simulink model "AxleSplitHEVv6_modif4"  (R2017a)
settings: Solver=ode5  StartTime=0.0  StopTime=400  FixedStep=hev_dt  MaxStep=0.01  RelTol=1e-3  AbsTol=1e-3  EnableMultiTasking=on
PostLoadFcn:
  | load('AxelSplitHEVv4_NEDC_18_06_15.mat')
values from neighbouring files (symbols this model uses):
  cmd_equivalent_conso_coef = 0.11126984    [AxelSplitHEVv4_NEDC_18_06_15.mat]
  cmd_qmax = 42    [AxelSplitHEVv4_NEDC_18_06_15.mat]
  cmd_specific_volume_l_per_g = 0.00133333333333    [AxelSplitHEVv4_NEDC_18_06_15.mat]
  dri_cycle_speed_sp = [0 0 0 4.16666667 4.16666667 2.777777778 0 0 0 4.166666667 4.166666667 8.88888889 ... (135 elements, 135x1)]    [AxelSplitHEVv4_NEDC_18_06_15.mat]
  dri_cycle_speed_time = [0 6 11 15 23 25 28 44 49 54 56 61 ... (135 elements, 135x1)]    [AxelSplitHEVv4_NEDC_18_06_15.mat]
  dri_gbx_sp = [0 1 0 1 2 0 1 2 3 2 0 1 ... (52 elements, 52x1)]    [AxelSplitHEVv4_NEDC_18_06_15.mat]
  dri_gbx_time = [0 11 25 49 55 93 117 123 134 177 185 206 ... (52 elements, 52x1)]    [AxelSplitHEVv4_NEDC_18_06_15.mat]
  dri_ki = 24.5    [AxelSplitHEVv4_NEDC_18_06_15.mat]
  dri_kp = 609    [AxelSplitHEVv4_NEDC_18_06_15.mat]
  fa_clu_pos = [1 1 0.7 0.5 0.3 0 0]    [AxelSplitHEVv4_NEDC_18_06_15.mat]
  fa_clu_pv = [0 0.1 0.3 0.5 0.7 0.9 1]    [AxelSplitHEVv4_NEDC_18_06_15.mat]
  fa_conso_idle = 0.153611111111    [AxelSplitHEVv4_NEDC_18_06_15.mat]
  fa_conso_speed = [200 300 400 500 600 700 800 900 1000 1100 1200 1300 ... (56 elements, 1x56)]    [AxelSplitHEVv4_NEDC_18_06_15.mat]
  fa_conso_torque = [0 6.66666666667 13.3333333333 20 26.6666666667 33.3333333333 40 46.6666666667 53.3333333333 60 66.6666666667 73.3333333333 ... (43 elements, 1x43)]    [AxelSplitHEVv4_NEDC_18_06_15.mat]
  fa_delta_derating = 500    [AxelSplitHEVv4_NEDC_18_06_15.mat]
  fa_differential_ratio = FDR.fa_differential_ratio    [Algorithme_eff.m]    (also in AxelSplitHEVv4_NEDC_18_06_15.mat = 3.72; fa_differential_ratio.mat = 3.72)
  fa_fuel_consumption = [nan nan nan nan nan nan nan nan nan nan nan nan ... (2408 elements, 43x56)]    [AxelSplitHEVv4_NEDC_18_06_15.mat]    (also in Curve_fitting_conso.m = fa_fuel_consumption/max(max(fa_fuel_consumption)))
  fa_gearbox_efficiency = 0.92    [AxelSplitHEVv4_NEDC_18_06_15.mat]
  fa_gearbox_ratio = FGR.fa_gearbox_ratio    [Algorithme_eff.m]    (also in AxelSplitHEVv4_NEDC_18_06_15.mat = [0 3.98 2.21 1.47 1.1 0.89 0.75]; fa_gearbox_ratio.mat = [0 3.98 2.21 1.47 1.1 0.89 0.75])
  fa_high_derating_point = 5700    [AxelSplitHEVv4_NEDC_18_06_15.mat]
  fa_ice_inertia = 0.058    [AxelSplitHEVv4_NEDC_18_06_15.mat]
  fa_kp_idle_tr_off = 0.116198282851    [AxelSplitHEVv4_NEDC_18_06_15.mat]
  fa_kp_idle_tr_on = [1 0.8653 2.8063 6.3428 11.3274 17.3036 24.3665]    [AxelSplitHEVv4_NEDC_18_06_15.mat]
  fa_low_derating_point = 4000    [AxelSplitHEVv4_NEDC_18_06_15.mat]
  fa_max_tq_clu = 206    [AxelSplitHEVv4_NEDC_18_06_15.mat]
  fa_max_tq_ice = [0 220 233.333333333 240 246.666666667 253.333333333 253.333333333 253.333333333 260 260 266.666666667 266.666666667 ... (52 elements, 1x52)]    [AxelSplitHEVv4_NEDC_18_06_15.mat]
  fa_n_ice = [0 20 250 850 1000 1250 1500 1750 2000 2250 2500 3000 ... (18 elements, 1x18)]    [AxelSplitHEVv4_NEDC_18_06_15.mat]
  fa_starter_rpm = [0 10 20 30 40 50 60 70 80 90 100 110 ... (101 elements, 1x101)]    [AxelSplitHEVv4_NEDC_18_06_15.mat]
  fa_starter_tq = [24 24 24 24 23.3333333333 23.3333333333 23.3333333333 22.6666666667 22.6666666667 22 21.3333333333 20.6666666667 ... (101 elements, 1x101)]    [AxelSplitHEVv4_NEDC_18_06_15.mat]
  fa_tau_ice = 0.0333    [AxelSplitHEVv4_NEDC_18_06_15.mat]
  fa_taui_idle_tr_off = 0.0820482966067    [AxelSplitHEVv4_NEDC_18_06_15.mat]
  fa_taui_idle_tr_on = 0.194086623254    [AxelSplitHEVv4_NEDC_18_06_15.mat]
  fa_tq_loss = [0 -11 -10 -9 -9 -10 -11 -11 -12 -13 -14 -15 ... (18 elements, 1x18)]    [AxelSplitHEVv4_NEDC_18_06_15.mat]
  fa_tq_max_speed = [200 700 800 900 1000 1100 1200 1300 1400 1500 1600 1700 ... (52 elements, 1x52)]    [AxelSplitHEVv4_NEDC_18_06_15.mat]
  hev_dt = 0.01    [AxelSplitHEVv4_NEDC_18_06_15.mat]
  pla_csat = 1.2    [AxelSplitHEVv4_NEDC_18_06_15.mat]
  pla_equivalent_weight = 1250    [AxelSplitHEVv4_NEDC_18_06_15.mat]
  pla_f = 0.0035272    [AxelSplitHEVv4_NEDC_18_06_15.mat]
  pla_k = 0.0002318    [AxelSplitHEVv4_NEDC_18_06_15.mat]
  pla_kaero = 0.52992    [AxelSplitHEVv4_NEDC_18_06_15.mat]
  pla_max_f_brakes = 1000    [AxelSplitHEVv4_NEDC_18_06_15.mat]
  pla_wheel_radius = 0.314    [AxelSplitHEVv4_NEDC_18_06_15.mat]
  ra_electrical_machine_efficiency = [nan nan nan nan nan nan nan 91.3 91.3 91.3 91.5 91.3 ... (777 elements, 37x21)]    [AxelSplitHEVv4_NEDC_18_06_15.mat]
  ra_electrical_machine_speed = [-12000 -10800 -9600 -8400 -7200 -6000 -4800 -3600 -2400 -1200 0 1200 ... (21 elements, 1x21)]    [AxelSplitHEVv4_NEDC_18_06_15.mat]
  ra_electrical_machine_tau = 0.1    [AxelSplitHEVv4_NEDC_18_06_15.mat]
  ra_electrical_machine_torque = [-79.6460176991 -75.2212389381 -70.796460177 -66.3716814159 -61.9469026549 -57.5221238938 -53.0973451327 -48.6725663717 -44.2477876106 -39.8230088496 -35.3982300885 -30.9734513274 ... (37 elements, 1x37)]    [AxelSplitHEVv4_NEDC_18_06_15.mat]
  ra_em_max_tq = [39.8230088496 44.2477876106 53.0973451327 57.5221238938 70.796460177 79.6460176991 79.6460176991 79.6460176991 79.6460176991 79.6460176991 79.6460176991 79.6460176991 ... (21 elements, 1x21)]    [AxelSplitHEVv4_NEDC_18_06_15.mat]
  ra_em_min_tq = [-39.8230088496 -44.2477876106 -53.0973451327 -57.5221238938 -70.796460177 -79.6460176991 -79.6460176991 -79.6460176991 -79.6460176991 -79.6460176991 -79.6460176991 -79.6460176991 ... (21 elements, 1x21)]    [AxelSplitHEVv4_NEDC_18_06_15.mat]
  ra_transmission_efficiency = 0.92    [AxelSplitHEVv4_NEDC_18_06_15.mat]
  reducteur = 2    [Main_modif.m]
  syse_aux_current = 33.3    [AxelSplitHEVv4_NEDC_18_06_15.mat]
  syse_aux_voltage = 12    [AxelSplitHEVv4_NEDC_18_06_15.mat]
  syse_bat_nominal_capacity_as = 151200    [AxelSplitHEVv4_NEDC_18_06_15.mat]
  syse_cdl = 5000    [AxelSplitHEVv4_NEDC_18_06_15.mat]
  syse_dcdc_efficency = [78 89.6 92.5 95.2 95 94.6]    [AxelSplitHEVv4_NEDC_18_06_15.mat]
  syse_dcdc_in_power = [54 135 202 405 1485 2000]    [AxelSplitHEVv4_NEDC_18_06_15.mat]
  syse_electrical_machine_torque_vs_power_speed_nneg = [38.4209635438 42.3166718474 53.0973451327 53.8788373627 63.500986907 77.9700595469 78.3175021924 76.9635177026 72.2987813984 47.9837613501 38.4209635438 42.3166718474 ... (220 elements, 10x22)]    [AxelSplitHEVv4_NEDC_18_06_15.mat]
  syse_electrical_machine_torque_vs_power_speed_npos = [-72.2987813984 -76.9635177026 -78.3175021924 -77.9700595469 -63.500986907 -53.8788373627 -53.0973451327 -42.3166718474 -38.4209635438 -72.2987813984 -76.9635177026 -78.3175021924 ... (198 elements, 9x22)]    [AxelSplitHEVv4_NEDC_18_06_15.mat]
  syse_em_in_power = [-49.1089315336 -44.1089315336 -39.1089315336 -34.1089315336 -29.1089315336 -24.1089315336 -19.1089315336 -14.1089315336 -9.10893153364 -4.10893153364 0.891068466363 5.89106846636 ... (22 elements, 1x22)]    [AxelSplitHEVv4_NEDC_18_06_15.mat]
  syse_max_charge_current = [8.4 8.4 42 92.4 92.4 92.4 92.4 92.4 79.8 42 21 4.2]    [AxelSplitHEVv4_NEDC_18_06_15.mat]
  syse_max_discharge_current = [42 42 79.8 159.6 180.6 180.6 180.6 180.6 180.6 180.6 180.6 180.6]    [AxelSplitHEVv4_NEDC_18_06_15.mat]
  syse_nb_cell = 52    [AxelSplitHEVv4_NEDC_18_06_15.mat]
  syse_rdl = 0.004    [AxelSplitHEVv4_NEDC_18_06_15.mat]
  syse_rser = 0.002    [AxelSplitHEVv4_NEDC_18_06_15.mat]
  syse_soc_current_limits = [0 10 20 20.1 30 40 50 60 70 80 90 100]    [AxelSplitHEVv4_NEDC_18_06_15.mat]
  syse_soc_initial = 0.8    [AxelSplitHEVv4_NEDC_18_06_15.mat]
  syse_soc_ocv = [0 5 10 20 40 50 60 70 80 90 100]    [AxelSplitHEVv4_NEDC_18_06_15.mat]
  syse_vocv = [2.5 3.2135 3.5127 3.66 3.7771 3.8181 3.8686 3.8978 3.9429 4.0006 4.198]    [AxelSplitHEVv4_NEDC_18_06_15.mat]
undefined symbols (not defined in the file or in its folder): DiscIntNeverNeededParam
libraries: simulink x23, simulink_extras x1
(part 3 of 3)

== system AxleSplitHEVv6_modif4/HEV model/Command/Torque repartition/Optimization Algorithm /Sfunction: Optimization Algorithm 32bits ==
  T : Inport
  V : Inport  Port=2
  Tmax_elec : Inport  Port=3
  Tmin_elec : Inport  Port=4
  Tmax_therm : Inport  Port=5
  Tmin_therm : Inport  Port=6
  GBX : Inport  Port=7
  SOC : Inport  Port=8
  MATLAB Function: Optimization Algorithm_sfcn : S-Function  FunctionName=MATLAB_sf  SFunctionModules=""  SFunctionDeploymentMode=off  EnableBusSupport=off  mask{rtw_sf_name=MATLAB_sf, showVar=off}
      mask prompts: rtw_sf_name "Simulink:masks:GenSFuncName_MP"; showVar "Simulink:masks:GenSFuncShowModuleList_MP"
      mask help: Simulink:masks:GenSFuncDesc_MD
      mask init:
      | displist = '';
      | if ~strcmp(get_param(gcb, 'FunctionName'), rtw_sf_name);
      |   set_param(gcb, 'FunctionName', rtw_sf_name);
      | end
      | % Check if we are generating code
      | rtw_mode = false;
      | if strcmpi(get_param(bdroot(gcb),'SimulationStatus'),'Initializing')
      | 	rtw_mode = strcmpi(get_param(bdroot(gcb),'BuildingRTWCode'),'on') && ...
      | 		~strcmpi(get_param(bdroot(gcb),'TargetStyle'),'SimulationTarget');
      | end
      | if showVar || rtw_mode
      | 	if exist('rtwsfunc') == 2 | exist('rtwsfunc') == 6
      | 		tmplist = rtwsfunc(rtw_sf_name,gcb);
      | 		tmplist = DAStudio.message('Simulink:masks:GenSFuncListOfModules_IC', tmplist);
      | 	elseif showVar
      | 		tmplist1 = DAStudio.message('Simulink:masks:GenSFuncListOfModules_IC', '');
      |         tmplist2 = DAStudio.message('Simulink:masks:GenSFuncNotLicensed_IC');
      |         tmplist = [tmplist1 tmplist2];
      |  	end
      | end
      | if showVar
      |   displist = tmplist;
      | end
      settings: CopyFcn=|
      | if ~strcmp(get_param(gcb,'Linkstatus'),'none') && ...
      | ~strcmp(get_param(gcb,'Linkstatus'),'implicit')
      |   set_param(gcb,'LinkStatus','none');
      | end
      mask Help: eval('feval(''rtwprivate'',''rtwhelpview'',''rtw_sfcn_block'')');
      mask Display:
      | port_label('input',1,'T');
      | port_label('input',2,'V');
      | port_label('input',3,'Tmax_elec');
      | port_label('input',4,'Tmin_elec');
      | port_label('input',5,'Tmax_therm');
      | port_label('input',6,'Tmin_therm');
      | port_label('input',7,'GBX');
      | port_label('input',8,'SOC');
      | port_label('output',1,'alpha_opt');
  __InputSSForSFun__ : Subsystem
  __OutputSSForSFun__ : Subsystem
  alpha_opt : Outport
  wires:
  T/1 -> __InputSSForSFun__/1(T)
  V/1 -> __InputSSForSFun__/2(V)
  Tmax_elec/1 -> __InputSSForSFun__/3(Tmax_elec)
  Tmin_elec/1 -> __InputSSForSFun__/4(Tmin_elec)
  Tmax_therm/1 -> __InputSSForSFun__/5(Tmax_therm)
  Tmin_therm/1 -> __InputSSForSFun__/6(Tmin_therm)
  GBX/1 -> __InputSSForSFun__/7(GBX)
  SOC/1 -> __InputSSForSFun__/8(SOC)
  __InputSSForSFun__/1(__UniqueOutportName__1__) -> MATLAB Function: Optimization Algorithm_sfcn/1
  __InputSSForSFun__/2(__UniqueOutportName__2__) -> MATLAB Function: Optimization Algorithm_sfcn/2
  __InputSSForSFun__/3(__UniqueOutportName__3__) -> MATLAB Function: Optimization Algorithm_sfcn/3
  __InputSSForSFun__/4(__UniqueOutportName__4__) -> MATLAB Function: Optimization Algorithm_sfcn/4
  __InputSSForSFun__/5(__UniqueOutportName__5__) -> MATLAB Function: Optimization Algorithm_sfcn/5
  __InputSSForSFun__/6(__UniqueOutportName__6__) -> MATLAB Function: Optimization Algorithm_sfcn/6
  __InputSSForSFun__/7(__UniqueOutportName__7__) -> MATLAB Function: Optimization Algorithm_sfcn/7
  __InputSSForSFun__/8(__UniqueOutportName__8__) -> MATLAB Function: Optimization Algorithm_sfcn/8
  MATLAB Function: Optimization Algorithm_sfcn/1 -> __OutputSSForSFun__/1(__UniqueInportName__1__)
  __OutputSSForSFun__/1(alpha_opt) -> alpha_opt/1

== system AxleSplitHEVv6_modif4/HEV model/Electrical system/Lithium-Ion Battery Management System/Battery model/li-ion Battery SOC ==
  SYSE_LIION_CURRENT : Inport
  Discrete-Time Integrator : DiscreteIntegrator  IntegratorMethod=Integration: Trapezoidal  InitialConditionSource=external  SampleTime=hev_dt  LimitOutput=on  UpperSaturationLimit=1  LowerSaturationLimit=0  ICPrevOutput=DiscIntNeverNeededParam  ICPrevScaledInput=DiscIntNeverNeededParam
  Divide1 : Product  Inputs=/*  SampleTime=hev_dt
  Gain : Gain  Gain=-1  SampleTime=hev_dt
  Nominal capacity : Constant  Value=syse_bat_nominal_capacity_as
  syse_soc_initial : Constant  Value=syse_soc_initial
  SYSE_SOC : Outport
  wires:
  Nominal capacity/1 -> Divide1/1  "A.s"
  Discrete-Time Integrator/1 -> SYSE_SOC/1
  syse_soc_initial/1 -> Discrete-Time Integrator/2
  Divide1/1 -> Discrete-Time Integrator/1  "s"
  SYSE_LIION_CURRENT/1 -> Gain/1  "A"
  Gain/1 -> Divide1/2

== system AxleSplitHEVv6_modif4/HEV model/Electrical system/Lithium-Ion Battery Management System/Battery model/li-ion battery voltage ==
  SYSE_SOC : Inport
  SYSE_LIION_CURRENT : Inport  Port=2
  Add2 : Sum  Inputs=+--  SampleTime=hev_dt
  Discrete Transfer Fcn1 : DiscreteTransferFcn  Numerator=[(hev_dt/(2*(syse_rdl*syse_cdl)+hev_dt)) (hev_dt/(2* (syse_rdl*syse_cdl)+hev_dt))]  Denominator=[1 ((hev_dt-2*(syse_rdl*syse_cdl)))/(2*(syse_rdl*syse_cdl)+hev_dt)]  SampleTime=hev_dt
  Gain : Gain  Gain=syse_rdl  SampleTime=hev_dt
  Lookup table Vocv : Lookup_n-D  NumberOfTableDimensions=1  BreakpointsForDimension1=syse_soc_ocv/100  Table=syse_vocv  SampleTime=hev_dt  RndMeth=Simplest  InputSameDT=on
  Rser : Gain  Gain=syse_rser  SampleTime=hev_dt
  nb of cell : Gain  Gain=syse_nb_cell  SampleTime=hev_dt
  SYSE_VOLTAGE_HV : Outport
  wires:
  SYSE_LIION_CURRENT/1 -> Gain/1, Rser/1
  SYSE_SOC/1 -> Lookup table Vocv/1
  Lookup table Vocv/1 -> Add2/1
  Add2/1 -> nb of cell/1
  nb of cell/1 -> SYSE_VOLTAGE_HV/1
  Rser/1 -> Add2/2
  Discrete Transfer Fcn1/1 -> Add2/3
  Gain/1 -> Discrete Transfer Fcn1/1

== system AxleSplitHEVv6_modif4/HEV model/Front Axle/CLUTCH/Clutch0/Stuck logic ==
  FA_W_CAR_INTEGRATOR_STATE : Inport
  FA_W_CAR : Inport  Port=2
  FA_TQ_ICE : Inport  Port=3
  FA_CLU_MAX_STATIC_TORQUE : Inport  Port=4
  Abs : Abs  SampleTime=hev_dt  SaturateOnIntegerOverflow=on
  Abs1 : Abs  SampleTime=hev_dt  SaturateOnIntegerOverflow=on
  Abs2 : Abs  SampleTime=hev_dt  SaturateOnIntegerOverflow=on
  Combinatorial Logic3 : CombinatorialLogic  Description=TRUTH_TABLE_FROM_FABIEN  TruthTable=[0;1;0;0;1;1;0;1]  SampleTime=hev_dt
  Compare To Constant : simulink/Logic and Bit Operations/Compare To Constant  relop=<=  const=40  OutDataTypeStr=boolean
  Delay : Delay  DelayLength=1  SampleTime=hev_dt
  Logic : Logic  IconShape=distinctive  SampleTime=hev_dt
  Mux : Mux  Inputs=3
  Relational Operator : RelationalOperator  Operator=<=  SampleTime=hev_dt  RndMeth=Nearest  InputSameDT=on
  Relational Operator1 : RelationalOperator  Operator=<=  SampleTime=hev_dt  RndMeth=Nearest  InputSameDT=on
  Scope2 : Scope
  Sum1 : Sum  Inputs=+-  SampleTime=hev_dt  SaturateOnIntegerOverflow=on  InputSameDT=on  OutDataTypeStr=Inherit: Same as first input
  FA_CLU_STUCK : Outport
  wires:
  FA_CLU_MAX_STATIC_TORQUE/1 -> Relational Operator1/2, Relational Operator/1
  Sum1/1 -> Abs2/1
  Abs1/1 -> Relational Operator1/1
  Delay/1 -> Mux/3
  Combinatorial Logic3/1 -> Delay/1, FA_CLU_STUCK/1
  Mux/1 -> Combinatorial Logic3/1
  Abs/1 -> Relational Operator/2
  Relational Operator/1 -> Mux/2
  Logic/1 -> Mux/1
  Abs2/1 -> Compare To Constant/1
  Compare To Constant/1 -> Logic/1
  Relational Operator1/1 -> Scope2/1, Logic/2
  FA_TQ_ICE/1 -> Abs1/1, Abs/1
  FA_W_CAR_INTEGRATOR_STATE/1 -> Sum1/1
  FA_W_CAR/1 -> Sum1/2

== system AxleSplitHEVv6_modif4/HEV model/Front Axle/CLUTCH/Clutch1/Stuck logic ==
  FA_W_CAR_INTEGRATOR_STATE : Inport
  FA_W_CAR : Inport  Port=2
  FA_TQ_ICE : Inport  Port=3
  FA_CLU_MAX_STATIC_TORQUE : Inport  Port=4
  Abs : Abs  SampleTime=hev_dt  SaturateOnIntegerOverflow=on
  Abs1 : Abs  SampleTime=hev_dt  SaturateOnIntegerOverflow=on
  Abs2 : Abs  SampleTime=hev_dt  SaturateOnIntegerOverflow=on
  Combinatorial Logic3 : CombinatorialLogic  Description=TRUTH_TABLE_FROM_FABIEN  TruthTable=[0;1;0;0;1;1;0;1]  SampleTime=hev_dt
  Compare To Constant : simulink/Logic and Bit Operations/Compare To Constant  relop=<=  const=40  OutDataTypeStr=boolean
  Delay : Delay  DelayLength=1  SampleTime=hev_dt
  Logic : Logic  IconShape=distinctive  SampleTime=hev_dt
  Mux : Mux  Inputs=3
  Relational Operator : RelationalOperator  Operator=<=  SampleTime=hev_dt  RndMeth=Nearest  InputSameDT=on
  Relational Operator1 : RelationalOperator  Operator=<=  SampleTime=hev_dt  RndMeth=Nearest  InputSameDT=on
  Scope2 : Scope
  Sum1 : Sum  Inputs=+-  SampleTime=hev_dt  SaturateOnIntegerOverflow=on  InputSameDT=on  OutDataTypeStr=Inherit: Same as first input
  FA_CLU_STUCK : Outport
  wires:
  FA_CLU_MAX_STATIC_TORQUE/1 -> Relational Operator1/2, Relational Operator/1
  Sum1/1 -> Abs2/1
  Abs1/1 -> Relational Operator1/1
  Delay/1 -> Mux/3
  Combinatorial Logic3/1 -> Delay/1, FA_CLU_STUCK/1
  Mux/1 -> Combinatorial Logic3/1
  Abs/1 -> Relational Operator/2
  Relational Operator/1 -> Mux/2
  Logic/1 -> Mux/1
  Abs2/1 -> Compare To Constant/1
  Compare To Constant/1 -> Logic/1
  Relational Operator1/1 -> Scope2/1, Logic/2
  FA_TQ_ICE/1 -> Abs1/1, Abs/1
  FA_W_CAR_INTEGRATOR_STATE/1 -> Sum1/1
  FA_W_CAR/1 -> Sum1/2

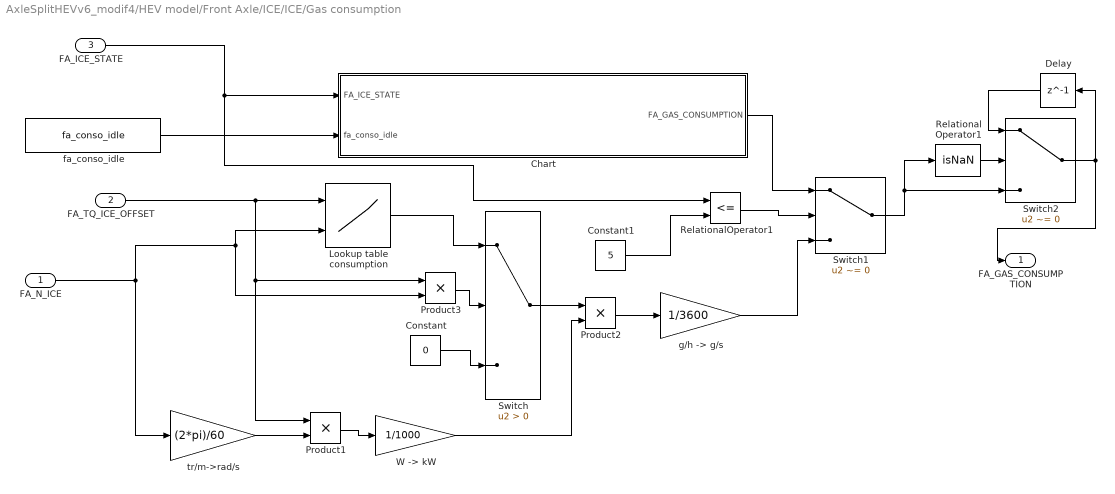
== system AxleSplitHEVv6_modif4/HEV model/Front Axle/ICE/ICE/Gas consumption ==
  FA_N_ICE : Inport
  FA_TQ_ICE_OFFSET : Inport  Port=2
  FA_ICE_STATE : Inport  Port=3
  Chart : Stateflow chart  TreatAsAtomicUnit=on
  Constant : Constant  Value=0
  Constant1 : Constant  Value=5
  Delay : Delay  DelayLength=1  SampleTime=hev_dt
  Lookup table consumption : Lookup_n-D  BreakpointsForDimension1=fa_conso_torque  BreakpointsForDimension2=fa_conso_speed  Table=fa_fuel_consumption  ExtrapMethod=Clip  UseLastTableValue=on  SampleTime=hev_dt  RndMeth=Simplest  InputSameDT=on
  Product1 : Product  SampleTime=hev_dt  RndMeth=Zero
  Product2 : Product  SampleTime=hev_dt  RndMeth=Zero
  Product3 : Product  SampleTime=hev_dt  RndMeth=Zero
  Relational Operator1 : RelationalOperator  Operator=isNaN  OutDataTypeStr=boolean  SampleTime=hev_dt  RndMeth=Nearest
  RelationalOperator1 : RelationalOperator  Operator=<=  OutDataTypeStr=boolean  SampleTime=hev_dt  RndMeth=Nearest
  Switch : Switch  Criteria=u2 > Threshold  SampleTime=hev_dt
  Switch1 : Switch  Criteria=u2 ~= 0  SampleTime=hev_dt
  Switch2 : Switch  Criteria=u2 ~= 0  SampleTime=hev_dt
  "W -> kW" : Gain  Gain=1/1000  SampleTime=hev_dt
  fa_conso_idle : Constant  Value=fa_conso_idle
  "g/h -> g/s" : Gain  Gain=1/3600  SampleTime=hev_dt
  tr/m->rad/s : Gain  Gain=(2*pi)/60  SampleTime=hev_dt
  FA_GAS_CONSUMPTION : Outport
  wires:
  Lookup table consumption/1 -> Switch/1
  Switch/1 -> Product2/1
  Constant/1 -> Switch/3
  "W -> kW"/1 -> Product2/2
  Product1/1 -> "W -> kW"/1
  tr/m->rad/s/1 -> Product1/2
  Product2/1 -> "g/h -> g/s"/1
  FA_N_ICE/1 -> Lookup table consumption/2, Product3/2, tr/m->rad/s/1
  FA_TQ_ICE_OFFSET/1 -> Product3/1, Product1/1, Lookup table consumption/1
  Product3/1 -> Switch/2
  Switch1/1 -> Switch2/3, Relational Operator1/1
  Switch2/1 -> FA_GAS_CONSUMPTION/1, Delay/1
  Relational Operator1/1 -> Switch2/2
  Delay/1 -> Switch2/1
  FA_ICE_STATE/1 -> RelationalOperator1/1, Chart/1(FA_ICE_STATE)
  "g/h -> g/s"/1 -> Switch1/3
  Chart/1(FA_GAS_CONSUMPTION) -> Switch1/1
  Constant1/1 -> RelationalOperator1/2
  RelationalOperator1/1 -> Switch1/2
  fa_conso_idle/1 -> Chart/2(fa_conso_idle)

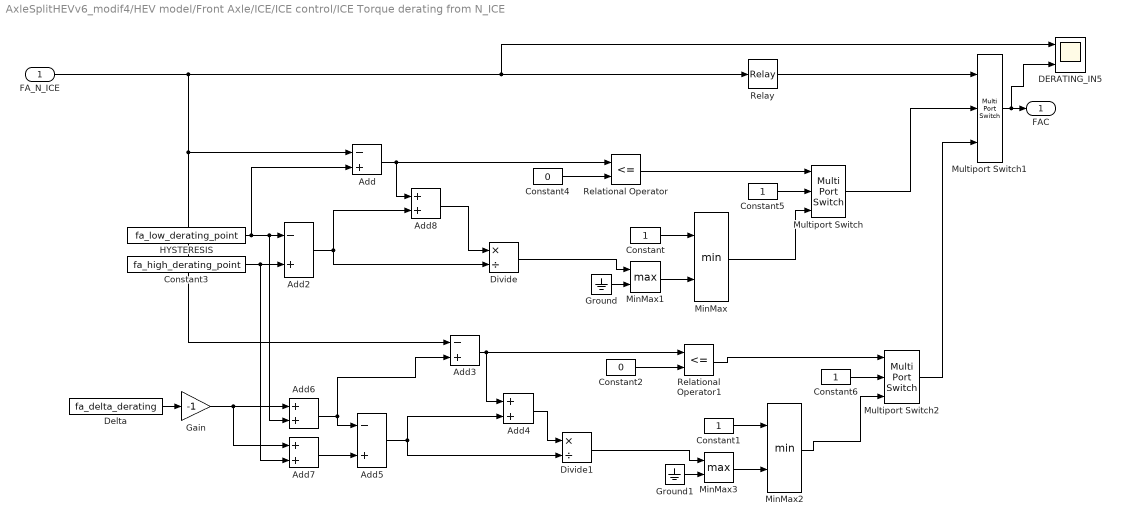
== system AxleSplitHEVv6_modif4/HEV model/Front Axle/ICE/ICE control/ICE Torque derating from N_ICE ==
  FA_N_ICE : Inport
  Add{,2..3,5} (4 alike) : Sum  Inputs=-+
  Add{4,6..8} (4 alike) : Sum
  Constant{,1,5..6} (4 alike) : Constant
  Constant2 : Constant  Value=0
  Constant3 : Constant  Value=fa_high_derating_point
  Constant4 : Constant  Value=0
  DERATING_IN5 : Scope  NumInputPorts=2
  Delta : Constant  Value=fa_delta_derating
  Divide : Product  Inputs=*/
  Divide1 : Product  Inputs=*/
  Gain : Gain  Gain=-1
  Ground : Ground
  Ground1 : Ground
  HYSTERESIS : Constant  Value=fa_low_derating_point
  MinMax : MinMax  Inputs=2
  MinMax1 : MinMax  Function=max  Inputs=2
  MinMax2 : MinMax  Inputs=2
  MinMax3 : MinMax  Function=max  Inputs=2
  Multiport Switch : MultiPortSwitch  DataPortOrder=Zero-based contiguous  Inputs=2
  Multiport Switch1 : MultiPortSwitch  DataPortOrder=Zero-based contiguous  Inputs=2
  Multiport Switch2 : MultiPortSwitch  DataPortOrder=Zero-based contiguous  Inputs=2
  Relational Operator : RelationalOperator  Operator=<=  OutDataTypeStr=boolean  RndMeth=Nearest
  Relational Operator1 : RelationalOperator  Operator=<=  OutDataTypeStr=boolean  RndMeth=Nearest
  Relay : Relay  OnSwitchValue=5750  OffSwitchValue=4900-500
  FAC : Outport
  wires:
  Gain/1 -> Add6/1, Add7/1
  Add4/1 -> Divide1/1
  Add8/1 -> Divide/1
  Add7/1 -> Add5/2
  Add6/1 -> Add3/2, Add5/1
  Constant6/1 -> Multiport Switch2/2
  MinMax2/1 -> Multiport Switch2/3
  Relational Operator1/1 -> Multiport Switch2/1
  Constant2/1 -> Relational Operator1/2
  Add3/1 -> Relational Operator1/1, Add4/1
  Divide1/1 -> MinMax3/1
  MinMax3/1 -> MinMax2/2
  Ground1/1 -> MinMax3/2
  Constant1/1 -> MinMax2/1
  FA_N_ICE/1 -> Add3/1, Add/1, Relay/1, DERATING_IN5/1
  Delta/1 -> Gain/1
  Constant3/1 -> Add2/2, Add7/2
  Multiport Switch2/1 -> Multiport Switch1/3
  HYSTERESIS/1 -> Add6/2, Add2/1, Add/2
  Multiport Switch/1 -> Multiport Switch1/2
  Constant5/1 -> Multiport Switch/2
  MinMax/1 -> Multiport Switch/3
  Relational Operator/1 -> Multiport Switch/1
  Constant4/1 -> Relational Operator/2
  Add/1 -> Add8/1, Relational Operator/1
  Relay/1 -> Multiport Switch1/1
  Divide/1 -> MinMax1/1
  MinMax1/1 -> MinMax/2
  Ground/1 -> MinMax1/2
  Constant/1 -> MinMax/1
  Multiport Switch1/1 -> FAC/1, DERATING_IN5/2
  Add2/1 -> Divide/2, Add8/2
  Add5/1 -> Divide1/2, Add4/2

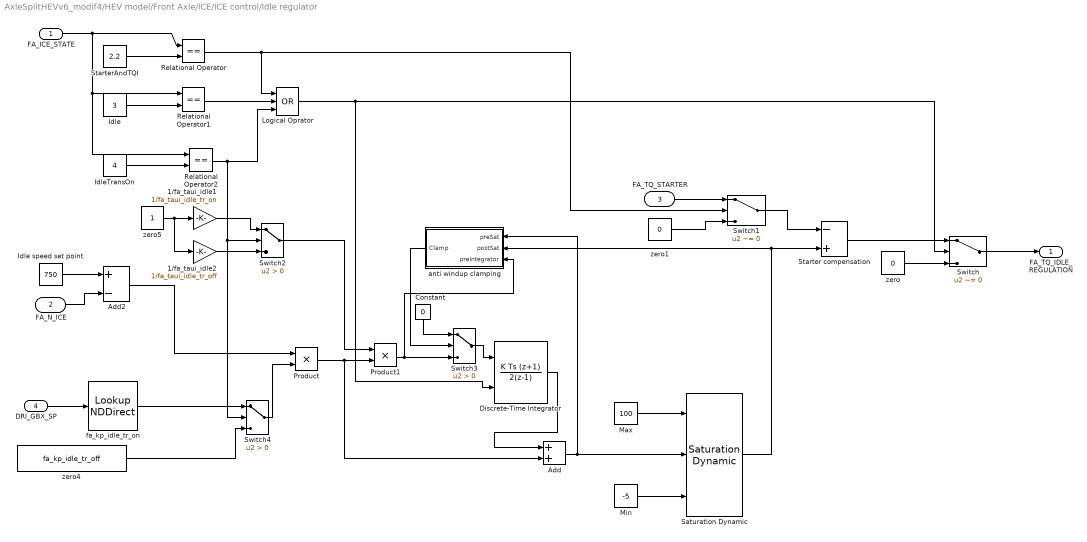
== system AxleSplitHEVv6_modif4/HEV model/Front Axle/ICE/ICE control/Idle regulator ==
  FA_ICE_STATE : Inport
  FA_N_ICE : Inport  Port=2
  FA_TQ_STARTER : Inport  Port=3
  DRI_GBX_SP : Inport  Port=4
  1/fa_taui_idle1 : Gain  Gain=1/fa_taui_idle_tr_on  SampleTime=hev_dt
  1/fa_taui_idle2 : Gain  Gain=1/fa_taui_idle_tr_off  SampleTime=hev_dt
  Add : Sum  SampleTime=hev_dt
  Add2 : Sum  Inputs=+-  SampleTime=hev_dt
  Constant : Constant  DisableCoverage=on  Value=0  OutDataTypeStr=Inherit: Inherit via back propagation  PreserveConstantTs=on
  Discrete-Time Integrator : DiscreteIntegrator  IntegratorMethod=Integration: Trapezoidal  ExternalReset=rising  SampleTime=hev_dt  ICPrevOutput=DiscIntNeverNeededParam  ICPrevScaledInput=DiscIntNeverNeededParam
  Idle : Constant  Value=3
  Idle speed set point : Constant  Value=750
  IdleTransOn : Constant  Value=4
  Logical Oprator : Logic  Operator=OR  Inputs=3  AllPortsSameDT=off  OutDataTypeStr=boolean  SampleTime=hev_dt
  Max : Constant  Value=100
  Min : Constant  Value=-5
  Product : Product  SampleTime=hev_dt  RndMeth=Zero
  Product1 : Product  SampleTime=hev_dt  RndMeth=Zero
  Relational Operator : RelationalOperator  Operator===  OutDataTypeStr=boolean  SampleTime=hev_dt  RndMeth=Nearest
  Relational Operator1 : RelationalOperator  Operator===  OutDataTypeStr=boolean  SampleTime=hev_dt  RndMeth=Nearest
  Relational Operator2 : RelationalOperator  Operator===  OutDataTypeStr=boolean  SampleTime=hev_dt  RndMeth=Nearest
  Saturation Dynamic : simulink/Discontinuities/Saturation Dynamic  OutMin=[]  OutMax=[]  OutDataTypeStr=Inherit: Same as second input  OutDataType=fixdt(1, 16)  OutScaling=2^-10  DoSatur=off
  Starter compensation : Sum  Inputs=-+  SampleTime=hev_dt
  StarterAndTQI : Constant  Value=2.2
  Switch : Switch  Criteria=u2 ~= 0  SampleTime=hev_dt
  Switch1 : Switch  Criteria=u2 ~= 0  SampleTime=hev_dt
  Switch2 : Switch  DisableCoverage=on  Criteria=u2 > Threshold  SampleTime=hev_dt  InputSameDT=on
  Switch3 : Switch  DisableCoverage=on  Criteria=u2 > Threshold  SampleTime=hev_dt  InputSameDT=on
  Switch4 : Switch  DisableCoverage=on  Criteria=u2 > Threshold  SampleTime=hev_dt  InputSameDT=on
  anti windup clamping : Subsystem
  fa_kp_idle_tr_on : LookupNDDirect  NumberOfTableDimensions=1  Table=fa_kp_idle_tr_on  SampleTime=hev_dt
  zero : Constant  Value=0
  zero1 : Constant  Value=0
  zero4 : Constant  Value=fa_kp_idle_tr_off
  zero5 : Constant
  FA_TQ_IDLE_REGULATION : Outport
  wires:
  FA_ICE_STATE/1 -> Relational Operator/1, Relational Operator1/1, Relational Operator2/1
  Switch/1 -> FA_TQ_IDLE_REGULATION/1
  zero/1 -> Switch/3
  Idle speed set point/1 -> Add2/1
  FA_N_ICE/1 -> Add2/2
  Relational Operator1/1 -> Logical Oprator/2
  StarterAndTQI/1 -> Relational Operator/2
  Idle/1 -> Relational Operator1/2
  zero1/1 -> Switch1/3
  FA_TQ_STARTER/1 -> Switch1/1
  IdleTransOn/1 -> Relational Operator2/2
  Starter compensation/1 -> Switch/1
  Logical Oprator/1 -> Switch/2, Discrete-Time Integrator/2
  anti windup clamping/1(Clamp) -> Switch3/2
  Constant/1 -> Switch3/1
  Product1/1 -> anti windup clamping/3(preIntegrator), Switch3/3
  zero5/1 -> 1/fa_taui_idle1/1, 1/fa_taui_idle2/1
  1/fa_taui_idle1/1 -> Switch2/1
  1/fa_taui_idle2/1 -> Switch2/3
  DRI_GBX_SP/1 -> fa_kp_idle_tr_on/1
  Product/1 -> Add/2, Product1/2
  Add2/1 -> Product/1
  fa_kp_idle_tr_on/1 -> Switch4/1
  Switch2/1 -> Product1/1
  zero4/1 -> Switch4/3
  Switch4/1 -> Product/2
  Relational Operator2/1 -> Logical Oprator/3, Switch4/2, Switch2/2
  Switch1/1 -> Starter compensation/1
  Discrete-Time Integrator/1 -> Add/1
  Relational Operator/1 -> Switch1/2, Logical Oprator/1
  Switch3/1 -> Discrete-Time Integrator/1
  Min/1 -> Saturation Dynamic/3
  Max/1 -> Saturation Dynamic/1
  Add/1 -> Saturation Dynamic/2, anti windup clamping/1(preSat)
  Saturation Dynamic/1 -> Starter compensation/2, anti windup clamping/2(postSat)

== system AxleSplitHEVv6_modif4/HEV model/Front Axle/ICE/ICE control/Injection shutdown ==
  FA_ICE_STATE : Inport
  CMD_FA_TQ_SP : Inport  Port=2
  PUC : Constant  Value=5.2
  Rate Limiter : RateLimiter  RisingSlewLimit=20  FallingSlewLimit=-100  SampleTimeMode=inherited
  Relational Operator1 : RelationalOperator  Operator===  OutDataTypeStr=boolean  SampleTime=hev_dt  RndMeth=Nearest
  Switch : Switch  Criteria=u2 ~= 0  SampleTime=hev_dt
  zero : Constant  Value=0
  FA_TQ_SP_INJECTION_OFF : Outport
  wires:
  Relational Operator1/1 -> Switch/2
  Rate Limiter/1 -> Switch/1
  FA_ICE_STATE/1 -> Relational Operator1/1
  CMD_FA_TQ_SP/1 -> Rate Limiter/1
  PUC/1 -> Relational Operator1/2
  Switch/1 -> FA_TQ_SP_INJECTION_OFF/1
  zero/1 -> Switch/3

== system AxleSplitHEVv6_modif4/HEV model/Front Axle/ICE/ICE control/Loss compentation ==
  FA_ICE_STATE : Inport
  FA_TQ_MIN_ICE : Inport  Port=2
  Logical Operator : Logic  AllPortsSameDT=off  OutDataTypeStr=boolean  SampleTime=hev_dt
  Loss compentation : UnaryMinus  SampleTime=hev_dt
  Relational Operator : RelationalOperator  Operator=~=  OutDataTypeStr=boolean  SampleTime=hev_dt  RndMeth=Nearest
  Relational Operator1 : RelationalOperator  Operator=~=  OutDataTypeStr=boolean  SampleTime=hev_dt  RndMeth=Nearest
  Stall : Constant
  Starter : Constant  Value=2.1
  Switch : Switch  Criteria=u2 ~= 0  SampleTime=hev_dt
  zero : Constant  Value=0
  FA_TQ_SP : Outport
  wires:
  FA_TQ_MIN_ICE/1 -> Switch/1
  zero/1 -> Switch/3
  Switch/1 -> Loss compentation/1
  Stall/1 -> Relational Operator1/2
  Starter/1 -> Relational Operator/2
  FA_ICE_STATE/1 -> Relational Operator/1, Relational Operator1/1
  Relational Operator/1 -> Logical Operator/1
  Relational Operator1/1 -> Logical Operator/2
  Loss compentation/1 -> FA_TQ_SP/1
  Logical Operator/1 -> Switch/2

== system AxleSplitHEVv6_modif4/HEV model/Front Axle/ICE/ICE control/Starter request ==
  FA_ICE_STATE : Inport
  Logical Operator : Logic  Operator=OR  AllPortsSameDT=off  OutDataTypeStr=boolean  SampleTime=hev_dt
  Relational Operator : RelationalOperator  Operator===  OutDataTypeStr=boolean  SampleTime=hev_dt  RndMeth=Nearest
  Relational Operator1 : RelationalOperator  Operator===  OutDataTypeStr=boolean  SampleTime=hev_dt  RndMeth=Nearest
  Starter : Constant  Value=2.1
  StarterAndTQI : Constant  Value=2.2
  FA_STARTER_REQUEST : Outport
  wires:
  Relational Operator1/1 -> Logical Operator/2
  Relational Operator/1 -> Logical Operator/1
  FA_ICE_STATE/1 -> Relational Operator1/1, Relational Operator/1
  StarterAndTQI/1 -> Relational Operator/2
  Starter/1 -> Relational Operator1/2
  Logical Operator/1 -> FA_STARTER_REQUEST/1

== system AxleSplitHEVv6_modif4/HEV model/Front Axle/ICE/ICE control/TopCrank for start ==
  FA_STARTER_REQUEST : Inport
  FA_N_ICE : Inport  Port=2
  FA_ICE_RESET_SYNCHRO : Inport  Port=3
  Delay : Delay  DelayLength=1  SampleTime=hev_dt
  Delay1 : Delay  DelayLength=1  SampleTime=hev_dt
  Detect Decrease : simulink/Logic and Bit Operations/Detect Decrease  vinit=0.0  InputProcessing=Inherited  OutDataTypeStr=uint8
  Discrete-Time Integrator : DiscreteIntegrator  IntegratorMethod=Integration: Trapezoidal  ExternalReset=rising  SampleTime=hev_dt  ICPrevOutput=DiscIntNeverNeededParam  ICPrevScaledInput=DiscIntNeverNeededParam
  Logical Operator : Logic  Operator=OR  AllPortsSameDT=off  OutDataTypeStr=boolean  SampleTime=hev_dt
  Logical Operator1 : Logic  AllPortsSameDT=off  OutDataTypeStr=boolean  SampleTime=hev_dt
  Logical Operator2 : Logic  Operator=NOT  AllPortsSameDT=off  OutDataTypeStr=boolean  SampleTime=hev_dt
  Math Function : Math  Operator=mod  SampleTime=hev_dt  SaturateOnIntegerOverflow=on
  top after 1.5 turn : Constant  Value=360*1.5
  tr/min > deg/s : Gain  Gain=6  SampleTime=hev_dt
  FA_ICE_SYNCHRO : Outport
  wires:
  tr/min > deg/s/1 -> Discrete-Time Integrator/1
  Discrete-Time Integrator/1 -> Math Function/1
  top after 1.5 turn/1 -> Math Function/2
  Math Function/1 -> Detect Decrease/1
  Detect Decrease/1 -> Delay/1
  FA_N_ICE/1 -> tr/min > deg/s/1
  FA_STARTER_REQUEST/1 -> Discrete-Time Integrator/2
  Logical Operator/1 -> Logical Operator1/1
  FA_ICE_RESET_SYNCHRO/1 -> Logical Operator2/1
  Logical Operator2/1 -> Logical Operator1/2
  Delay1/1 -> Logical Operator/1
  Logical Operator1/1 -> Delay1/1, FA_ICE_SYNCHRO/1
  Delay/1 -> Logical Operator/2

== system AxleSplitHEVv6_modif4/HEV model/Front Axle/ICE/ICE control/Transfer of the command ==
  FA_ICE_STATE : Inport
  CMD_FA_TQ_SP : Inport  Port=2
  Force traking : Constant  Value=5.1  VectorParams1D=off
  Force traking1 : Constant  Value=3  VectorParams1D=off
  IdleTransOn : Constant  Value=4
  Logical Operator : Logic  Operator=OR  Inputs=3  AllPortsSameDT=off  OutDataTypeStr=boolean  SampleTime=hev_dt
  Relational Operator : RelationalOperator  Operator===  OutDataTypeStr=boolean  SampleTime=hev_dt  RndMeth=Nearest
  Relational Operator1 : RelationalOperator  Operator===  OutDataTypeStr=boolean  SampleTime=hev_dt  RndMeth=Nearest
  Relational Operator2 : RelationalOperator  Operator===  OutDataTypeStr=boolean  SampleTime=hev_dt  RndMeth=Nearest
  Switch : Switch  Criteria=u2 ~= 0  SampleTime=hev_dt
  zero : Constant  Value=0
  FA_TQ_SP : Outport
  wires:
  Relational Operator1/1 -> Logical Operator/2
  Relational Operator/1 -> Logical Operator/1
  FA_ICE_STATE/1 -> Relational Operator/1, Relational Operator1/1, Relational Operator2/1
  IdleTransOn/1 -> Relational Operator/2
  Force traking/1 -> Relational Operator1/2
  Logical Operator/1 -> Switch/2
  Switch/1 -> FA_TQ_SP/1
  zero/1 -> Switch/3
  CMD_FA_TQ_SP/1 -> Switch/1
  Force traking1/1 -> Relational Operator2/2
  Relational Operator2/1 -> Logical Operator/3

== system AxleSplitHEVv6_modif4/HEV model/Command/Torque repartition/Optimization Algorithm /Sfunction: Optimization Algorithm 32bits/__InputSSForSFun__ ==
  T : Inport
  V : Inport  Port=2
  Tmax_elec : Inport  Port=3
  Tmin_elec : Inport  Port=4
  Tmax_therm : Inport  Port=5
  Tmin_therm : Inport  Port=6
  GBX : Inport  Port=7
  SOC : Inport  Port=8
  __UniqueOutportName__1__ : Outport
  __UniqueOutportName__2__ : Outport  Port=2
  __UniqueOutportName__3__ : Outport  Port=3
  __UniqueOutportName__4__ : Outport  Port=4
  __UniqueOutportName__5__ : Outport  Port=5
  __UniqueOutportName__6__ : Outport  Port=6
  __UniqueOutportName__7__ : Outport  Port=7
  __UniqueOutportName__8__ : Outport  Port=8
  wires:
  T/1 -> __UniqueOutportName__1__/1
  V/1 -> __UniqueOutportName__2__/1
  Tmax_elec/1 -> __UniqueOutportName__3__/1
  Tmin_elec/1 -> __UniqueOutportName__4__/1
  Tmax_therm/1 -> __UniqueOutportName__5__/1
  Tmin_therm/1 -> __UniqueOutportName__6__/1
  GBX/1 -> __UniqueOutportName__7__/1
  SOC/1 -> __UniqueOutportName__8__/1

== system AxleSplitHEVv6_modif4/HEV model/Command/Torque repartition/Optimization Algorithm /Sfunction: Optimization Algorithm 32bits/__OutputSSForSFun__ ==
  __UniqueInportName__1__ : Inport
  alpha_opt : Outport
  wires:
  __UniqueInportName__1__/1 -> alpha_opt/1  "alpha_opt"

== system AxleSplitHEVv6_modif4/HEV model/Front Axle/ICE/ICE control/Idle regulator/anti windup clamping ==
  preSat : Inport
  postSat : Inport  Port=2
  preIntegrator : Inport  Port=3
  AND : Logic  DisableCoverage=on  OutDataTypeStr=boolean  SampleTime=hev_dt
  Delay : Delay  DelayLength=1  SampleTime=hev_dt
  Equal : RelationalOperator  DisableCoverage=on  Operator===  OutDataTypeStr=boolean  SampleTime=hev_dt  RndMeth=Nearest  InputSameDT=on
  NotEqual : RelationalOperator  DisableCoverage=on  Operator=~=  OutDataTypeStr=boolean  SampleTime=hev_dt  RndMeth=Nearest  InputSameDT=on
  SignPreIntegrator : Signum  DisableCoverage=on  SampleTime=hev_dt
  SignPreSat : Signum  DisableCoverage=on  SampleTime=hev_dt
  Clamp : Outport
  wires:
  preSat/1 -> SignPreSat/1, NotEqual/1
  postSat/1 -> NotEqual/2
  preIntegrator/1 -> SignPreIntegrator/1
  SignPreSat/1 -> Equal/1
  NotEqual/1 -> AND/1
  SignPreIntegrator/1 -> Equal/2
  Equal/1 -> AND/2
  AND/1 -> Delay/1
  Delay/1 -> Clamp/1

== stateflow chart AxleSplitHEVv6_modif4/HEV model/Front Axle/ICE/ICE/Gas consumption/Chart ==
  state STATE_3
    du : FA_GAS_CONSUMPTION=fa_conso_idle;
  state STATE_5
    du : FA_GAS_CONSUMPTION=0;
  state STATE_22
    du : FA_GAS_CONSUMPTION=0;
  state STATE_4
    du : FA_GAS_CONSUMPTION=fa_conso_idle;
  state STATE_1
    du : FA_GAS_CONSUMPTION=0;
  state STATE_21
    du : FA_GAS_CONSUMPTION=0;
  STATE_1 -> STATE_5 [order 2] : [(FA_ICE_STATE==5)]
  STATE_22 -> STATE_5 [order 4] : [((FA_ICE_STATE==5.1)||(FA_ICE_STATE==5.2))]
  STATE_1 -> STATE_3 [order 4] : [(FA_ICE_STATE==3)]
  STATE_1 -> STATE_22 [order 3] : [(FA_ICE_STATE==2.2)]
  STATE_3 -> STATE_5 [order 3] : [((FA_ICE_STATE==5.1)||(FA_ICE_STATE==5.2))]
  STATE_22 -> STATE_4 [order 3] : [(FA_ICE_STATE==4)]
  (default) -> STATE_1
  STATE_22 -> STATE_3 [order 1] : [(FA_ICE_STATE==3)]
  STATE_4 -> STATE_3 [order 1] : [(FA_ICE_STATE==3)]
  STATE_21 -> STATE_22 [order 2] : [(FA_ICE_STATE==2.2)]
  STATE_4 -> STATE_5 [order 2] : [((FA_ICE_STATE==5.1)||(FA_ICE_STATE==5.2))]
  STATE_21 -> STATE_1 [order 1] : [(FA_ICE_STATE==1)]
  STATE_3 -> STATE_4 [order 1] : [(FA_ICE_STATE==4)]
  STATE_5 -> STATE_4 [order 1] : [(FA_ICE_STATE==4)]
  STATE_1 -> STATE_21 [order 1] : [(FA_ICE_STATE==2.1)]
  STATE_3 -> STATE_22 [order 4] : [(FA_ICE_STATE==2)]
  STATE_5 -> STATE_1 [order 2] : [(FA_ICE_STATE==1)]
  STATE_5 -> STATE_3 [order 3] : [(FA_ICE_STATE==3)]
  STATE_22 -> STATE_1 [order 2] : [(FA_ICE_STATE==1)]
  STATE_3 -> STATE_21 [order 5] : [(FA_ICE_STATE==2.1)]
  STATE_4 -> STATE_21 [order 4] : [(FA_ICE_STATE==2.1)]
  STATE_4 -> STATE_1 [order 3] : [(FA_ICE_STATE==1)]
  STATE_3 -> STATE_1 [order 2] : [(FA_ICE_STATE==1)]
  data: FA_GAS_CONSUMPTION output; FA_ICE_STATE input; fa_conso_idle input

== stateflow chart AxleSplitHEVv6_modif4/HEV model/Front Axle/ICE/ICE control/ICE state machine ==
  state Start
    state Starter
      en: FA_ICE_STATE=2.1;
    state StarterAndTQI
      en: FA_ICE_STATE=2.2;
    (default) -> Starter
    Starter -> StarterAndTQI : [(FA_N_ICE>250)&&(FA_ICE_SYNCHRO==1)]
  state Stall
    en: FA_ICE_STATE=1;
  state Running
    state Idle
      en: FA_ICE_STATE=3;
    state IdleTransOn
      en: FA_ICE_STATE=4;
    state Force_tracking
      state Standard_force_tracking
        en: FA_ICE_STATE=5.1;
      state InjectionInhibed
        en: FA_ICE_STATE=5.2;
      (default) -> Standard_force_tracking
      InjectionInhibed -> Standard_force_tracking [order 1] : [CMD_FA_TQ_SP>FA_TQ_MIN_ICE]
      Standard_force_tracking -> InjectionInhibed : [(CMD_FA_TQ_SP==FA_TQ_MIN_ICE)]
    (default) -> (junction 111)
    (junction 111) -> IdleTransOn [order 1] : [(FA_CLU_STUCK!=0)&&(DRI_GBX_SP!=0)]
    (junction 111) -> Idle [order 2]
    IdleTransOn -> Idle [order 1] : [((FA_CLU_STUCK==0)||(DRI_GBX_SP==0))]
    Idle -> IdleTransOn : [(FA_CLU_STUCK!=0)&&(DRI_GBX_SP!=0)]
    Force_tracking -> Idle : [((FA_CLU_STUCK==0)||(DRI_GBX_SP==0))]
    IdleTransOn -> Force_tracking [order 2] : [(FA_CLU_STUCK==1)&&(DRI_GBX_SP!=0)&&(CMD_FA_TQ_SP>0)]
    InjectionInhibed -> IdleTransOn [order 2] : [(FA_N_ICE<1200)&&(FA_CLU_STUCK==1)&&(DRI_GBX_SP!=0)]
  (default) -> Stall
  Start -> Stall [order 2] : [FA_START_ICE!=1]
  Stall -> Start [order 1] : [(FA_START_ICE==1)&&(FA_N_ICE<30)]
  Stall -> Force_tracking [order 2] : [(FA_START_ICE==1)&&(FA_N_ICE>600)&&(DRI_GBX_SP!=0)&&(FA_CLU_STUCK==1)]
  Running -> Stall : [(FA_START_ICE!=1)||(FA_N_ICE<400)]
  StarterAndTQI -> Stall : [(FA_N_ICE<250)]
  Start -> Running [order 1] : [FA_N_ICE>600]
  data: FA_ICE_SYNCHRO input; FA_N_ICE input double; CMD_FA_TQ_SP input double; DRI_GBX_SP input double; FA_ICE_STATE output double; FA_CLU_STUCK input; FA_TQ_MIN_ICE input double; FA_START_ICE input double

== stateflow chart AxleSplitHEVv6_modif4/HEV model/Driver1/Clutch command/Clutch Command/SHIFT DOWN ==
  state First_state
    entry: output_memory = 1;
  state Second_state
    entry: output_memory = 0;
  (default) -> (junction 11)
  (junction 11) -> First_state [order 1] : [last_DRI_REF_GBX > DRI_REF_GBX]
  (junction 11) -> Second_state [order 2] : [DRI_REF_GBX == actual_DRI_GBX]
  First_state -> Second_state : [DRI_REF_GBX == actual_DRI_GBX]
  Second_state -> First_state : [last_DRI_REF_GBX > DRI_REF_GBX]
  data: output_memory output; last_DRI_REF_GBX input; DRI_REF_GBX input; actual_DRI_GBX input

== stateflow chart AxleSplitHEVv6_modif4/HEV model/Command/Start_Stop/START//STOP 1 ==
  state WAKEUP
    entry:ENERGY_MANAGEMENT_ON_OFF=0;
  state RUNNING
    entry: ENERGY_MANAGEMENT_ON_OFF=1;
    entry: FA_START_ICE=0;
    state START
      entry: FA_START_ICE=1;
      k = 0;
      during : k = k+1;
      exit : k = 0;
    state STOP
      entry: FA_START_ICE=0;
    STOP -> START : [(CMD_START_STOP ==0)]
    (default) -> STOP
    START -> STOP : [(CMD_START_STOP ==1)&&(k >200)]
  note: In the state START , we don't allowing a use of the ICE for less than 2 seconds
  (default) -> WAKEUP
  RUNNING -> WAKEUP : [(START == 0)]
  WAKEUP -> RUNNING : [(START == 1)]
  data: START input; CMD_START_STOP input; FA_START_ICE output; ENERGY_MANAGEMENT_ON_OFF output; k local

== stateflow chart AxleSplitHEVv6_modif4/HEV model/Driver1/Clutch command/Clutch Command/SHIFT UP ==
  state First_state
    entry: output_memory = 1;
  state Second_state
    entry: output_memory = 0;
  (default) -> (junction 11)
  (junction 11) -> First_state [order 1] : [last_DRI_REF_GBX < DRI_REF_GBX]
  (junction 11) -> Second_state [order 2] : [DRI_REF_GBX == actual_DRI_GBX]
  First_state -> Second_state : [DRI_REF_GBX == actual_DRI_GBX]
  Second_state -> First_state : [last_DRI_REF_GBX < DRI_REF_GBX]
  data: output_memory output; last_DRI_REF_GBX input; DRI_REF_GBX input; actual_DRI_GBX input
